simulink library "Library_Drivetrain"  (R2020b)
settings: Solver=VariableStepAuto  StartTime=0.0  StopTime=10.0  RelTol=1e-3
undefined symbols (not defined in the file or in its folder): DrivetrainLeft, DrivetrainRight
libraries: simulink x18, mbd_s32k1xx_ec_toolbox x8
(part 1 of 2)
settings Model: Creator=cbeal  LastModifiedBy=cbeal

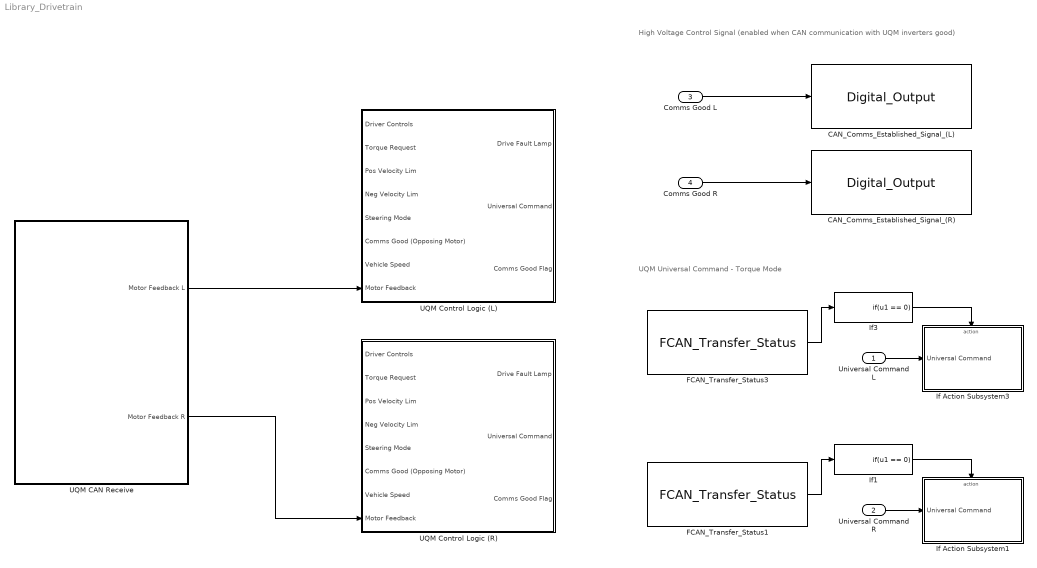
== system Library_Drivetrain ==
  note: UQM Universal Command - Torque Mode
  note: High Voltage Control Signal
      | (enabled when CAN communication with UQM inverters good)
  Universal Command L : Inport
  Universal Command R : Inport  Port=2
  Comms Good L : Inport  Port=3
  Comms Good R : Inport  Port=4
  CAN_Comms_Established_Signal_(L) : mbd_s32k1xx_ec_toolbox/GPIO Blocks/Digital_Output  gpio_pin=PTD8: [PTD8 | Port D I/O]  init_val=Low  drive_strength=Low
  CAN_Comms_Established_Signal_(R) : mbd_s32k1xx_ec_toolbox/GPIO Blocks/Digital_Output  gpio_pin=PTE15: [PTE15 | Port E I/O]  init_val=Low  drive_strength=Low
  FCAN_Transfer_Status1 : mbd_s32k1xx_ec_toolbox/Communication Blocks/CAN Blocks/FCAN_Transfer_Status  can_instance=1  can_mb_idx=4
  FCAN_Transfer_Status3 : mbd_s32k1xx_ec_toolbox/Communication Blocks/CAN Blocks/FCAN_Transfer_Status  can_instance=1  can_mb_idx=3
  If Action Subsystem1 : Subsystem  TreatAsAtomicUnit=on
  If Action Subsystem3 : Subsystem  TreatAsAtomicUnit=on
  If1 : If  IfExpression=u1 == 0  ShowElse=off
  If3 : If  IfExpression=u1 == 0  ShowElse=off
  UQM CAN Receive : Subsystem
  UQM Control Logic (L) : Subsystem  TreatAsAtomicUnit=on
      settings: RTWSystemCode=Inline
  UQM Control Logic (R) : Subsystem  TreatAsAtomicUnit=on
      settings: RTWSystemCode=Inline
  wires:
  UQM CAN Receive/1(Motor Feedback L) -> UQM Control Logic (L)/8(Motor Feedback)
  UQM CAN Receive/2(Motor Feedback R) -> UQM Control Logic (R)/8(Motor Feedback)
  Universal Command L/1 -> If Action Subsystem3/1(Universal Command)
  Universal Command R/1 -> If Action Subsystem1/1(Universal Command)
  If1/1 -> If Action Subsystem1/Action
  If3/1 -> If Action Subsystem3/Action
  FCAN_Transfer_Status3/1 -> If3/1
  FCAN_Transfer_Status1/1 -> If1/1
  Comms Good R/1 -> CAN_Comms_Established_Signal_(R)/1
  Comms Good L/1 -> CAN_Comms_Established_Signal_(L)/1

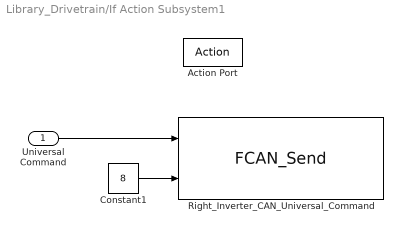
== system Library_Drivetrain/If Action Subsystem1 ==
  Universal Command : Inport
  Action Port : ActionPort  ActionPortLabel=if(u1 == 0)
  Constant1 : Constant  Value=8  OutDataTypeStr=Inherit: Inherit via back propagation
  Right_Inverter_CAN_Universal_Command : mbd_s32k1xx_ec_toolbox/Communication Blocks/CAN Blocks/FCAN_Send  can_instance=1  can_mode=Non-blocking  can_timeout_ms=0  can_mb_idx=4  can_extended_id=off  can_is_remote=off  can_id=F5  show_adv_opts=off  can_fd_enable=off  can_enable_brs=off  can_fd_padding=0
  wires:
  Constant1/1 -> Right_Inverter_CAN_Universal_Command/2
  Universal Command/1 -> Right_Inverter_CAN_Universal_Command/1

== system Library_Drivetrain/If Action Subsystem3 ==
  Universal Command : Inport
  Action Port : ActionPort  ActionPortLabel=if(u1 == 0)
  Constant1 : Constant  Value=8  OutDataTypeStr=Inherit: Inherit via back propagation
  Left_Inverter_CAN_Universal_Command : mbd_s32k1xx_ec_toolbox/Communication Blocks/CAN Blocks/FCAN_Send  can_instance=1  can_mode=Non-blocking  can_timeout_ms=0  can_mb_idx=3  can_extended_id=off  can_is_remote=off  can_id=85  show_adv_opts=off  can_fd_enable=off  can_enable_brs=off  can_fd_padding=0
  wires:
  Universal Command/1 -> Left_Inverter_CAN_Universal_Command/1
  Constant1/1 -> Left_Inverter_CAN_Universal_Command/2

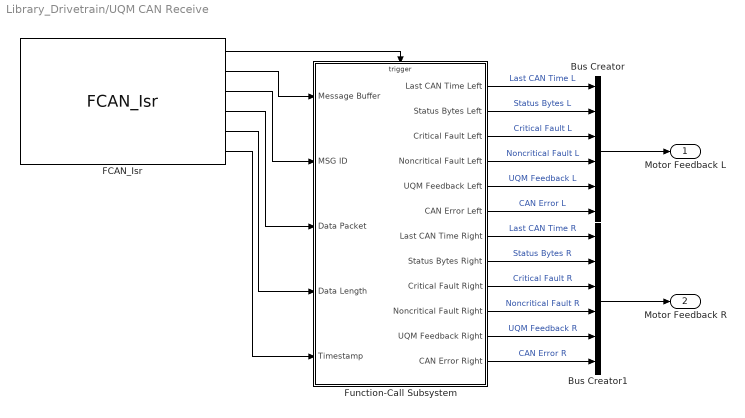
== system Library_Drivetrain/UQM CAN Receive ==
  Bus Creator : BusCreator  Inputs=6
  Bus Creator1 : BusCreator  Inputs=6
  FCAN_Isr : mbd_s32k1xx_ec_toolbox/Communication Blocks/CAN Blocks/FCAN_Isr  can_instance=1  can_event=Rx Complete
  Function-Call Subsystem : Subsystem  TreatAsAtomicUnit=on
  Motor Feedback L : Outport
  Motor Feedback R : Outport  Port=2
  wires:
  FCAN_Isr/2 -> Function-Call Subsystem/1(Message Buffer)
  FCAN_Isr/5 -> Function-Call Subsystem/4(Data Length)
  FCAN_Isr/4 -> Function-Call Subsystem/3(Data Packet)
  FCAN_Isr/3 -> Function-Call Subsystem/2(MSG ID)
  FCAN_Isr/1 -> Function-Call Subsystem/Trigger
  FCAN_Isr/6 -> Function-Call Subsystem/5(Timestamp)
  Function-Call Subsystem/1(Last CAN Time Left) -> Bus Creator/1  "Last CAN Time L"
  Function-Call Subsystem/2(Status Bytes Left) -> Bus Creator/2  "Status Bytes L"
  Function-Call Subsystem/3(Critical Fault Left) -> Bus Creator/3  "Critical Fault L"
  Function-Call Subsystem/4(Noncritical Fault Left) -> Bus Creator/4  "Noncritical Fault L"
  Function-Call Subsystem/5(UQM Feedback Left) -> Bus Creator/5  "UQM Feedback L"
  Function-Call Subsystem/6(CAN Error Left) -> Bus Creator/6  "CAN Error L"
  Bus Creator/1 -> Motor Feedback L/1
  Function-Call Subsystem/7(Last CAN Time Right) -> Bus Creator1/1  "Last CAN Time R"
  Function-Call Subsystem/8(Status Bytes Right) -> Bus Creator1/2  "Status Bytes R"
  Function-Call Subsystem/9(Critical Fault Right) -> Bus Creator1/3  "Critical Fault R"
  Function-Call Subsystem/10(Noncritical Fault Right) -> Bus Creator1/4  "Noncritical Fault R"
  Function-Call Subsystem/11(UQM Feedback Right) -> Bus Creator1/5  "UQM Feedback R"
  Function-Call Subsystem/12(CAN Error Right) -> Bus Creator1/6  "CAN Error R"
  Bus Creator1/1 -> Motor Feedback R/1

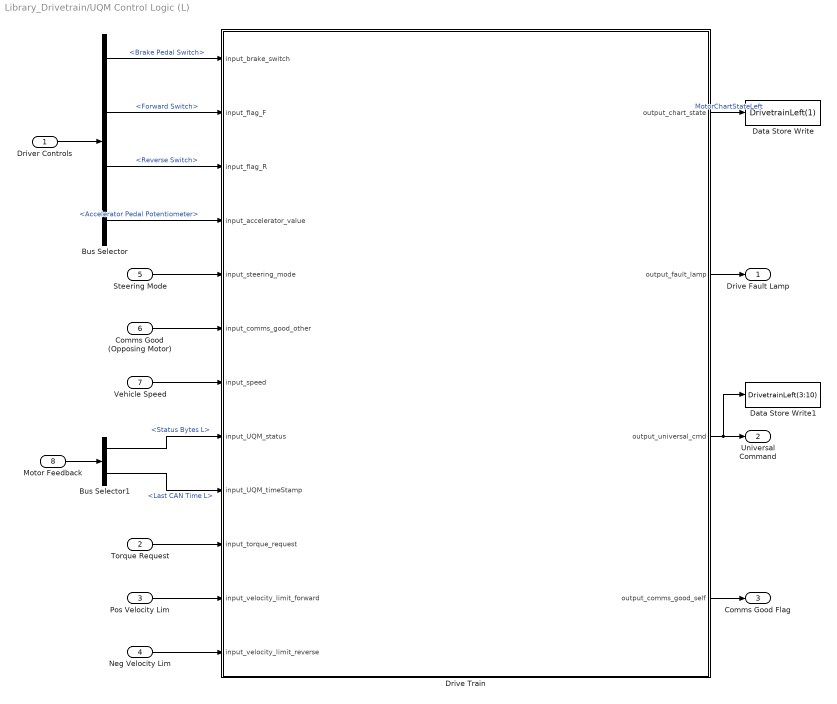
== system Library_Drivetrain/UQM Control Logic (L) ==
  Driver Controls : Inport
  Torque Request : Inport  Port=2
  Pos Velocity Lim : Inport  Port=3
  Neg Velocity Lim : Inport  Port=4
  Steering Mode : Inport  Port=5
  Comms Good (Opposing Motor) : Inport  Port=6
  Vehicle Speed : Inport  Port=7
  Motor Feedback : Inport  Port=8
  Bus Selector : BusSelector  OutputSignals=Brake Pedal Switch,Forward Switch,Reverse Switch,Accelerator Pedal Potentiometer
  Bus Selector1 : BusSelector  OutputSignals=Status Bytes L,Last CAN Time L
  Data Store Write : DataStoreWrite  DataStoreName=DrivetrainLeft  DataStoreElements=DrivetrainLeft(1)
  Data Store Write1 : DataStoreWrite  DataStoreName=DrivetrainLeft  DataStoreElements=DrivetrainLeft(3:10)
  Drive Train : Stateflow chart  TreatAsAtomicUnit=on
      settings: RTWSystemCode=Inline  PortSchema="{\"entries\":[{\"content\":{\"sides\":[{\"content\":{\"connectorIds\":[\"In1\",\"In6\",\"In7\",\"In5\",\"In3\",\"In2\",\"In4\",\"In8\",\"In9\",\"In10\",\"In11\",\"In12\"]},\"type\":\"ConnectorPlacement.EquallySpacedRectSide\",\"uuid\":\"177131f9-522e-4b0e-bcb9-1c7f9e428ff0\"},{\"content\":{\"connectorIds\":[\"Out1\",\"Out2\",\"Out3\",\"Out4\"],\"side\":\"RIGHT\"},\"type\":\"ConnectorPlacement.EquallySpacedRectSide\",\"uuid\":\"9c682759-a653-4ffd-ae7a-9eeda4cc7cea\"},{\"content\":{\"connectorIds\":[],\"side\":\"TOP\"},\"type\":\"ConnectorPlacement.EquallySpacedRectSide\",\"uuid\":\"64c937ee-85b6-4d66-9bbf-f706f379c6d1\"},{\"content\":{\"connectorIds\":[],\"side\":\"HIDDEN\"},\"type\":\"ConnectorPlacement.EquallySpacedRectSide\",\"uuid\":\"ab261037-f33d-4213-8477-31b1a1e7b9c4\"}]},\"type\":\"ConnectorPlacement.EquallySpacedConnector\",\"uuid\":\"dccf0cbc-1b8f-4706-82c8-4b900e553059\"}],\"packageUris\":[\"http://schema.mathworks.com/mf0/Connector/R2020b\"],\"version\":\"1.0\"}"
  Drive Fault Lamp : Outport
  Universal Command : Outport  Port=2
  Comms Good Flag : Outport  Port=3
  wires:
  Drive Train/1(output_chart_state) -> Data Store Write/1  "MotorChartStateLeft"
  Drive Train/3(output_universal_cmd) -> Data Store Write1/1, Universal Command/1
  Drive Train/4(output_comms_good_self) -> Comms Good Flag/1
  Drive Train/2(output_fault_lamp) -> Drive Fault Lamp/1
  Driver Controls/1 -> Bus Selector/1
  Bus Selector/2 -> Drive Train/6(input_flag_F)  "<Forward Switch>"
  Bus Selector/3 -> Drive Train/7(input_flag_R)  "<Reverse Switch>"
  Bus Selector/1 -> Drive Train/1(input_brake_switch)  "<Brake Pedal Switch>"
  Bus Selector/4 -> Drive Train/5(input_accelerator_value)  "<Accelerator Pedal Potentiometer>"
  Torque Request/1 -> Drive Train/10(input_torque_request)
  Pos Velocity Lim/1 -> Drive Train/11(input_velocity_limit_forward)
  Neg Velocity Lim/1 -> Drive Train/12(input_velocity_limit_reverse)
  Steering Mode/1 -> Drive Train/3(input_steering_mode)
  Comms Good (Opposing Motor)/1 -> Drive Train/2(input_comms_good_other)
  Vehicle Speed/1 -> Drive Train/4(input_speed)
  Bus Selector1/2 -> Drive Train/9(input_UQM_timeStamp)  "<Last CAN Time L>"
  Bus Selector1/1 -> Drive Train/8(input_UQM_status)  "<Status Bytes L>"
  Motor Feedback/1 -> Bus Selector1/1

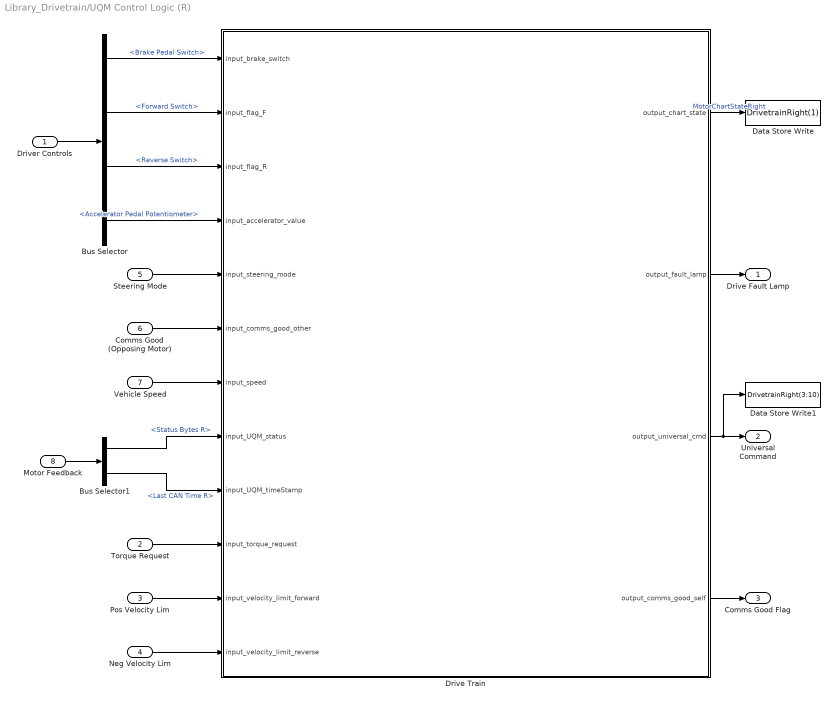
== system Library_Drivetrain/UQM Control Logic (R) ==
  Driver Controls : Inport
  Torque Request : Inport  Port=2
  Pos Velocity Lim : Inport  Port=3
  Neg Velocity Lim : Inport  Port=4
  Steering Mode : Inport  Port=5
  Comms Good (Opposing Motor) : Inport  Port=6
  Vehicle Speed : Inport  Port=7
  Motor Feedback : Inport  Port=8
  Bus Selector : BusSelector  OutputSignals=Brake Pedal Switch,Forward Switch,Reverse Switch,Accelerator Pedal Potentiometer
  Bus Selector1 : BusSelector  OutputSignals=Status Bytes R,Last CAN Time R
  Data Store Write : DataStoreWrite  DataStoreName=DrivetrainRight  DataStoreElements=DrivetrainRight(1)
  Data Store Write1 : DataStoreWrite  DataStoreName=DrivetrainRight  DataStoreElements=DrivetrainRight(3:10)
  Drive Train : Stateflow chart  TreatAsAtomicUnit=on
      settings: RTWSystemCode=Inline  PortSchema="{\"entries\":[{\"content\":{\"sides\":[{\"content\":{\"connectorIds\":[\"In1\",\"In6\",\"In7\",\"In5\",\"In3\",\"In2\",\"In4\",\"In8\",\"In9\",\"In10\",\"In11\",\"In12\"]},\"type\":\"ConnectorPlacement.EquallySpacedRectSide\",\"uuid\":\"177131f9-522e-4b0e-bcb9-1c7f9e428ff0\"},{\"content\":{\"connectorIds\":[\"Out1\",\"Out2\",\"Out3\",\"Out4\"],\"side\":\"RIGHT\"},\"type\":\"ConnectorPlacement.EquallySpacedRectSide\",\"uuid\":\"9c682759-a653-4ffd-ae7a-9eeda4cc7cea\"},{\"content\":{\"connectorIds\":[],\"side\":\"TOP\"},\"type\":\"ConnectorPlacement.EquallySpacedRectSide\",\"uuid\":\"64c937ee-85b6-4d66-9bbf-f706f379c6d1\"},{\"content\":{\"connectorIds\":[],\"side\":\"HIDDEN\"},\"type\":\"ConnectorPlacement.EquallySpacedRectSide\",\"uuid\":\"ab261037-f33d-4213-8477-31b1a1e7b9c4\"}]},\"type\":\"ConnectorPlacement.EquallySpacedConnector\",\"uuid\":\"dccf0cbc-1b8f-4706-82c8-4b900e553059\"}],\"packageUris\":[\"http://schema.mathworks.com/mf0/Connector/R2020b\"],\"version\":\"1.0\"}"
  Drive Fault Lamp : Outport
  Universal Command : Outport  Port=2
  Comms Good Flag : Outport  Port=3
  wires:
  Motor Feedback/1 -> Bus Selector1/1
  Bus Selector1/1 -> Drive Train/8(input_UQM_status)  "<Status Bytes R>"
  Bus Selector1/2 -> Drive Train/9(input_UQM_timeStamp)  "<Last CAN Time R>"
  Vehicle Speed/1 -> Drive Train/4(input_speed)
  Comms Good (Opposing Motor)/1 -> Drive Train/2(input_comms_good_other)
  Steering Mode/1 -> Drive Train/3(input_steering_mode)
  Neg Velocity Lim/1 -> Drive Train/12(input_velocity_limit_reverse)
  Pos Velocity Lim/1 -> Drive Train/11(input_velocity_limit_forward)
  Torque Request/1 -> Drive Train/10(input_torque_request)
  Bus Selector/4 -> Drive Train/5(input_accelerator_value)  "<Accelerator Pedal Potentiometer>"
  Bus Selector/1 -> Drive Train/1(input_brake_switch)  "<Brake Pedal Switch>"
  Bus Selector/3 -> Drive Train/7(input_flag_R)  "<Reverse Switch>"
  Bus Selector/2 -> Drive Train/6(input_flag_F)  "<Forward Switch>"
  Driver Controls/1 -> Bus Selector/1
  Drive Train/2(output_fault_lamp) -> Drive Fault Lamp/1
  Drive Train/4(output_comms_good_self) -> Comms Good Flag/1
  Drive Train/3(output_universal_cmd) -> Universal Command/1, Data Store Write1/1
  Drive Train/1(output_chart_state) -> Data Store Write/1  "MotorChartStateRight"

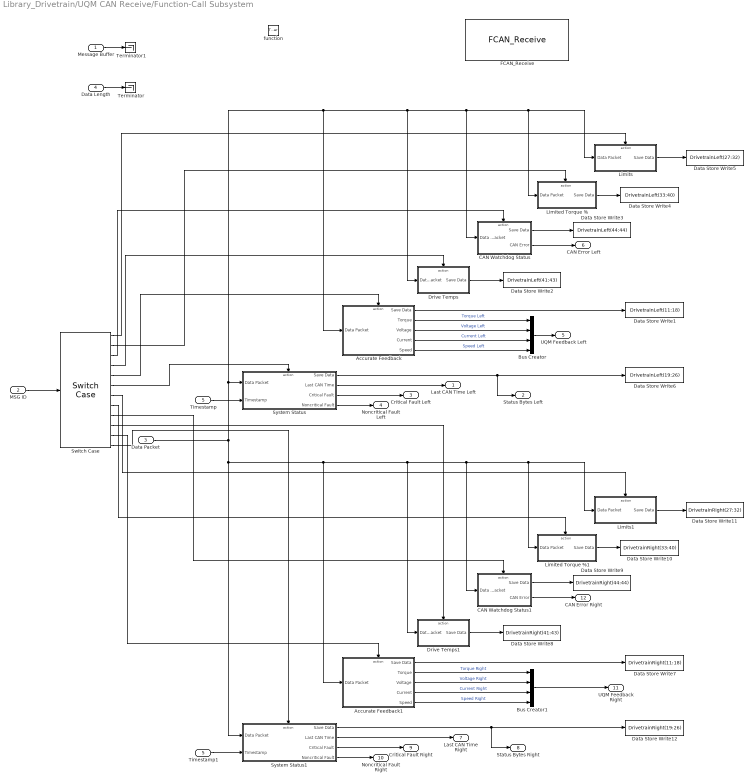
== system Library_Drivetrain/UQM CAN Receive/Function-Call Subsystem ==
  Message Buffer : Inport
  MSG ID : Inport  Port=2
  Data Packet : Inport  Port=3
  Data Length : Inport  Port=4
  Timestamp : Inport  Port=5
  function : TriggerPort  TriggerType=function-call  VariantControl=Variant
  Accurate Feedback : Subsystem  TreatAsAtomicUnit=on
      settings: RTWSystemCode=Inline
  Accurate Feedback1 : Subsystem  TreatAsAtomicUnit=on
      settings: RTWSystemCode=Inline
  Bus Creator : BusCreator  Inputs=4
  Bus Creator1 : BusCreator  Inputs=4
  CAN Watchdog Status : Subsystem  TreatAsAtomicUnit=on
      settings: RTWSystemCode=Inline
  CAN Watchdog Status1 : Subsystem  TreatAsAtomicUnit=on
      settings: RTWSystemCode=Inline
  Data Store Write1 : DataStoreWrite  DataStoreName=DrivetrainLeft  DataStoreElements=DrivetrainLeft(11:18)
  Data Store Write10 : DataStoreWrite  DataStoreName=DrivetrainRight  DataStoreElements=DrivetrainRight(33:40)
  Data Store Write11 : DataStoreWrite  DataStoreName=DrivetrainRight  DataStoreElements=DrivetrainRight(27:32)
  Data Store Write12 : DataStoreWrite  DataStoreName=DrivetrainRight  DataStoreElements=DrivetrainRight(19:26)
  Data Store Write2 : DataStoreWrite  DataStoreName=DrivetrainLeft  DataStoreElements=DrivetrainLeft(41:43)
  Data Store Write3 : DataStoreWrite  DataStoreName=DrivetrainLeft  DataStoreElements=DrivetrainLeft(44:44)
  Data Store Write4 : DataStoreWrite  DataStoreName=DrivetrainLeft  DataStoreElements=DrivetrainLeft(33:40)
  Data Store Write5 : DataStoreWrite  DataStoreName=DrivetrainLeft  DataStoreElements=DrivetrainLeft(27:32)
  Data Store Write6 : DataStoreWrite  DataStoreName=DrivetrainLeft  DataStoreElements=DrivetrainLeft(19:26)
  Data Store Write7 : DataStoreWrite  DataStoreName=DrivetrainRight  DataStoreElements=DrivetrainRight(11:18)
  Data Store Write8 : DataStoreWrite  DataStoreName=DrivetrainRight  DataStoreElements=DrivetrainRight(41:43)
  Data Store Write9 : DataStoreWrite  DataStoreName=DrivetrainRight  DataStoreElements=DrivetrainRight(44:44)
  Drive Temps : Subsystem  TreatAsAtomicUnit=on
      settings: RTWSystemCode=Inline
  Drive Temps1 : Subsystem  TreatAsAtomicUnit=on
      settings: RTWSystemCode=Inline
  FCAN_Receive : mbd_s32k1xx_ec_toolbox/Communication Blocks/CAN Blocks/FCAN_Receive  can_instance=1  can_mode=Non-blocking  can_timeout_ms=0  can_mb_idx=0  can_extended_id=off  can_is_remote=off  can_id=0  can_msg_mask=0  show_adv_opts=off  can_use_rxfifo=off  can_fd_enable=off
  Limited Torque % : Subsystem  TreatAsAtomicUnit=on
      settings: RTWSystemCode=Inline
  Limited Torque %1 : Subsystem  TreatAsAtomicUnit=on
      settings: RTWSystemCode=Inline
  Limits : Subsystem  TreatAsAtomicUnit=on
      settings: RTWSystemCode=Inline
  Limits1 : Subsystem  TreatAsAtomicUnit=on
      settings: RTWSystemCode=Inline
  Switch Case : SwitchCase  CaseConditions={hex2dec('8C'),hex2dec('8D'),hex2dec('8F'),hex2dec('8E'),hex2dec('89'),hex2dec('8A'),hex2dec('FC'),hex2dec('FD'),hex2dec('FF'),hex2dec('FE'),hex2dec('F9'),hex2dec('FA')}  ShowDefaultCase=off
  System Status : Subsystem  TreatAsAtomicUnit=on
      settings: RTWSystemCode=Inline
  System Status1 : Subsystem  TreatAsAtomicUnit=on
      settings: RTWSystemCode=Inline
  Terminator : Terminator
  Terminator1 : Terminator
  Timestamp1 : InportShadow  Port=5
  Last CAN Time Left : Outport
  Status Bytes Left : Outport  Port=2
  Critical Fault Left : Outport  Port=3
  Noncritical Fault Left : Outport  Port=4
  UQM Feedback Left : Outport  Port=5
  CAN Error Left : Outport  Port=6
  Last CAN Time Right : Outport  Port=7
  Status Bytes Right : Outport  Port=8
  Critical Fault Right : Outport  Port=9
  Noncritical Fault Right : Outport  Port=10
  UQM Feedback Right : Outport  Port=11
  CAN Error Right : Outport  Port=12
  wires:
  Drive Temps/1(Save Data) -> Data Store Write2/1
  CAN Watchdog Status/1(Save Data) -> Data Store Write3/1
  System Status/1(Save Data) -> Data Store Write6/1, Status Bytes Left/1
  Switch Case/2 -> Limited Torque %/Action
  Switch Case/4 -> Drive Temps/Action
  Switch Case/3 -> CAN Watchdog Status/Action
  Accurate Feedback/3(Voltage) -> Bus Creator/2  "Voltage Left"
  MSG ID/1 -> Switch Case/1
  Timestamp/1 -> System Status/2(Timestamp)
  System Status/4(Noncritical Fault) -> Noncritical Fault Left/1
  Message Buffer/1 -> Terminator1/1
  System Status/3(Critical Fault) -> Critical Fault Left/1
  CAN Watchdog Status/2(CAN Error) -> CAN Error Left/1
  Switch Case/1 -> Limits/Action
  Bus Creator/1 -> UQM Feedback Left/1
  Data Length/1 -> Terminator/1
  Switch Case/6 -> System Status/Action
  Accurate Feedback/5(Speed) -> Bus Creator/4  "Speed Left"
  Switch Case/5 -> Accurate Feedback/Action
  System Status/2(Last CAN Time) -> Last CAN Time Left/1
  Accurate Feedback/4(Current) -> Bus Creator/3  "Current Left"
  Limits/1(Save Data) -> Data Store Write5/1
  Accurate Feedback/1(Save Data) -> Data Store Write1/1
  Limited Torque %/1(Save Data) -> Data Store Write4/1
  Accurate Feedback/2(Torque) -> Bus Creator/1  "Torque Left"
  Limited Torque %1/1(Save Data) -> Data Store Write10/1
  Accurate Feedback1/2(Torque) -> Bus Creator1/1  "Torque Right"
  Accurate Feedback1/1(Save Data) -> Data Store Write7/1
  Limits1/1(Save Data) -> Data Store Write11/1
  System Status1/2(Last CAN Time) -> Last CAN Time Right/1
  Switch Case/12 -> System Status1/Action
  Switch Case/11 -> Accurate Feedback1/Action
  System Status1/3(Critical Fault) -> Critical Fault Right/1
  Data Packet/1 -> Accurate Feedback1/1(Data Packet), Drive Temps1/1(Data Packet), CAN Watchdog Status1/1(Data Packet), Limited Torque %1/1(Data Packet), Limits1/1(Data Packet), System Status1/1(Data Packet), Accurate Feedback/1(Data Packet), Drive Temps/1(Data Packet), CAN Watchdog Status/1(Data Packet), Limited Torque %/1(Data Packet), Limits/1(Data Packet), System Status/1(Data Packet)
  Bus Creator1/1 -> UQM Feedback Right/1
  Switch Case/10 -> Drive Temps1/Action
  Accurate Feedback1/4(Current) -> Bus Creator1/3  "Current Right"
  Switch Case/9 -> CAN Watchdog Status1/Action
  Accurate Feedback1/5(Speed) -> Bus Creator1/4  "Speed Right"
  Drive Temps1/1(Save Data) -> Data Store Write8/1
  CAN Watchdog Status1/1(Save Data) -> Data Store Write9/1
  System Status1/4(Noncritical Fault) -> Noncritical Fault Right/1
  System Status1/1(Save Data) -> Data Store Write12/1, Status Bytes Right/1
  Switch Case/7 -> Limits1/Action
  Accurate Feedback1/3(Voltage) -> Bus Creator1/2  "Voltage Right"
  Timestamp1/1 -> System Status1/2(Timestamp)
  Switch Case/8 -> Limited Torque %1/Action
  CAN Watchdog Status1/2(CAN Error) -> CAN Error Right/1

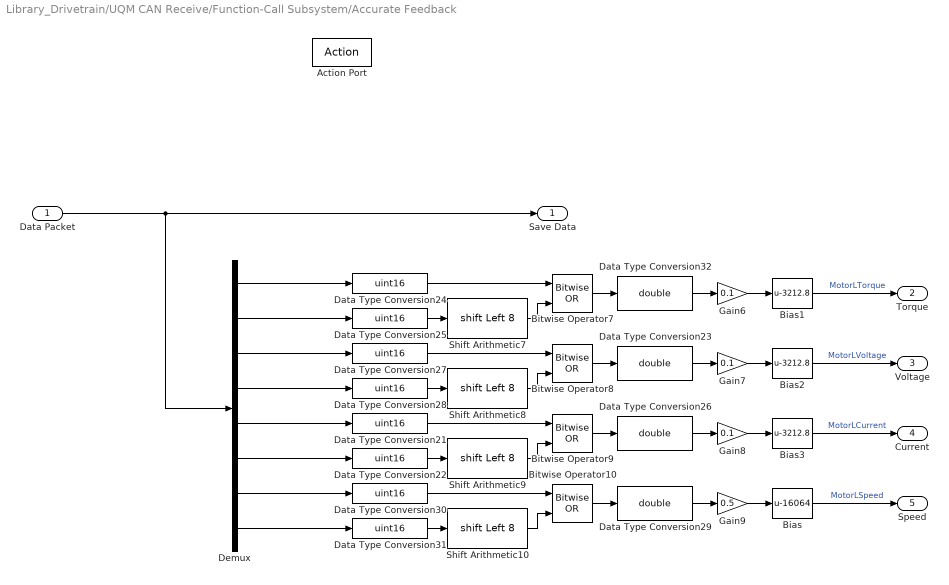
== system Library_Drivetrain/UQM CAN Receive/Function-Call Subsystem/Accurate Feedback ==
  Data Packet : Inport
  Action Port : ActionPort
  Bias : Bias  Bias=-16064
  Bias1 : Bias  Bias=-3212.8
  Bias2 : Bias  Bias=-3212.8
  Bias3 : Bias  Bias=-3212.8
  Bitwise Operator{7..10} (4 alike) : simulink/Logic and Bit Operations/Bitwise Operator  logicop=OR  UseBitMask=off  NumInputPorts=2  BitMask=bin2dec('11011001')  BitMaskRealWorld=Stored Integer
  Data Type Conversion{21..22,24..25,27..28,30..31} (8 alike) : DataTypeConversion  OutDataTypeStr=uint16
  Data Type Conversion{23,26,29,32} (4 alike) : DataTypeConversion  OutDataTypeStr=double
  Demux : Demux  Outputs=8
  Gain6 : Gain  Gain=0.1  OutDataTypeStr=Inherit: Inherit via back propagation
  Gain7 : Gain  Gain=0.1  OutDataTypeStr=Inherit: Inherit via back propagation
  Gain8 : Gain  Gain=0.1  OutDataTypeStr=Inherit: Inherit via back propagation
  Gain9 : Gain  Gain=0.5  OutDataTypeStr=Inherit: Inherit via back propagation
  Shift Arithmetic{7..10} (4 alike) : ArithShift  BitShiftNumber=8  BitShiftDirection=Left
  Save Data : Outport
  Torque : Outport  Port=2
  Voltage : Outport  Port=3
  Current : Outport  Port=4
  Speed : Outport  Port=5
  wires:
  Bias1/1 -> Torque/1  "MotorLTorque"
  Bias2/1 -> Voltage/1  "MotorLVoltage"
  Bias3/1 -> Current/1  "MotorLCurrent"
  Bias/1 -> Speed/1  "MotorLSpeed"
  Data Type Conversion24/1 -> Bitwise Operator7/1
  Gain7/1 -> Bias2/1
  Data Type Conversion30/1 -> Bitwise Operator10/1
  Data Type Conversion22/1 -> Shift Arithmetic9/1
  Data Type Conversion21/1 -> Bitwise Operator9/1
  Bitwise Operator9/1 -> Data Type Conversion26/1
  Gain9/1 -> Bias/1
  Data Type Conversion28/1 -> Shift Arithmetic8/1
  Data Type Conversion32/1 -> Gain6/1
  Shift Arithmetic7/1 -> Bitwise Operator7/2
  Gain8/1 -> Bias3/1
  Data Type Conversion26/1 -> Gain8/1
  Bitwise Operator10/1 -> Data Type Conversion29/1
  Bitwise Operator8/1 -> Data Type Conversion23/1
  Gain6/1 -> Bias1/1
  Shift Arithmetic10/1 -> Bitwise Operator10/2
  Data Type Conversion27/1 -> Bitwise Operator8/1
  Data Type Conversion29/1 -> Gain9/1
  Bitwise Operator7/1 -> Data Type Conversion32/1
  Data Type Conversion31/1 -> Shift Arithmetic10/1
  Data Type Conversion25/1 -> Shift Arithmetic7/1
  Shift Arithmetic8/1 -> Bitwise Operator8/2
  Shift Arithmetic9/1 -> Bitwise Operator9/2
  Data Type Conversion23/1 -> Gain7/1
  Demux/1 -> Data Type Conversion24/1
  Demux/2 -> Data Type Conversion25/1
  Demux/3 -> Data Type Conversion27/1
  Demux/4 -> Data Type Conversion28/1
  Demux/5 -> Data Type Conversion21/1
  Demux/6 -> Data Type Conversion22/1
  Demux/7 -> Data Type Conversion30/1
  Demux/8 -> Data Type Conversion31/1
  Data Packet/1 -> Demux/1, Save Data/1

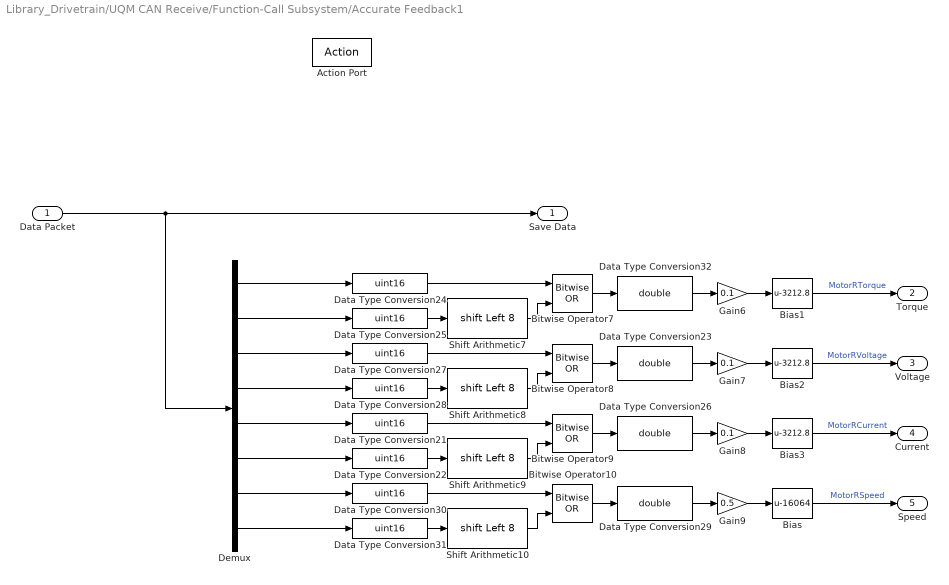
== system Library_Drivetrain/UQM CAN Receive/Function-Call Subsystem/Accurate Feedback1 ==
  Data Packet : Inport
  Action Port : ActionPort
  Bias : Bias  Bias=-16064
  Bias1 : Bias  Bias=-3212.8
  Bias2 : Bias  Bias=-3212.8
  Bias3 : Bias  Bias=-3212.8
  Bitwise Operator{7..10} (4 alike) : simulink/Logic and Bit Operations/Bitwise Operator  logicop=OR  UseBitMask=off  NumInputPorts=2  BitMask=bin2dec('11011001')  BitMaskRealWorld=Stored Integer
  Data Type Conversion{21..22,24..25,27..28,30..31} (8 alike) : DataTypeConversion  OutDataTypeStr=uint16
  Data Type Conversion{23,26,29,32} (4 alike) : DataTypeConversion  OutDataTypeStr=double
  Demux : Demux  Outputs=8
  Gain6 : Gain  Gain=0.1  OutDataTypeStr=Inherit: Inherit via back propagation
  Gain7 : Gain  Gain=0.1  OutDataTypeStr=Inherit: Inherit via back propagation
  Gain8 : Gain  Gain=0.1  OutDataTypeStr=Inherit: Inherit via back propagation
  Gain9 : Gain  Gain=0.5  OutDataTypeStr=Inherit: Inherit via back propagation
  Shift Arithmetic{7..10} (4 alike) : ArithShift  BitShiftNumber=8  BitShiftDirection=Left
  Save Data : Outport
  Torque : Outport  Port=2
  Voltage : Outport  Port=3
  Current : Outport  Port=4
  Speed : Outport  Port=5
  wires:
  Bias1/1 -> Torque/1  "MotorRTorque"
  Bias2/1 -> Voltage/1  "MotorRVoltage"
  Bias3/1 -> Current/1  "MotorRCurrent"
  Bias/1 -> Speed/1  "MotorRSpeed"
  Data Type Conversion24/1 -> Bitwise Operator7/1
  Gain7/1 -> Bias2/1
  Data Type Conversion30/1 -> Bitwise Operator10/1
  Data Type Conversion22/1 -> Shift Arithmetic9/1
  Data Type Conversion21/1 -> Bitwise Operator9/1
  Bitwise Operator9/1 -> Data Type Conversion26/1
  Gain9/1 -> Bias/1
  Data Type Conversion28/1 -> Shift Arithmetic8/1
  Data Type Conversion32/1 -> Gain6/1
  Shift Arithmetic7/1 -> Bitwise Operator7/2
  Gain8/1 -> Bias3/1
  Data Type Conversion26/1 -> Gain8/1
  Bitwise Operator10/1 -> Data Type Conversion29/1
  Bitwise Operator8/1 -> Data Type Conversion23/1
  Gain6/1 -> Bias1/1
  Shift Arithmetic10/1 -> Bitwise Operator10/2
  Data Type Conversion27/1 -> Bitwise Operator8/1
  Data Type Conversion29/1 -> Gain9/1
  Bitwise Operator7/1 -> Data Type Conversion32/1
  Data Type Conversion31/1 -> Shift Arithmetic10/1
  Data Type Conversion25/1 -> Shift Arithmetic7/1
  Shift Arithmetic8/1 -> Bitwise Operator8/2
  Shift Arithmetic9/1 -> Bitwise Operator9/2
  Data Type Conversion23/1 -> Gain7/1
  Demux/1 -> Data Type Conversion24/1
  Demux/2 -> Data Type Conversion25/1
  Demux/3 -> Data Type Conversion27/1
  Demux/4 -> Data Type Conversion28/1
  Demux/5 -> Data Type Conversion21/1
  Demux/6 -> Data Type Conversion22/1
  Demux/7 -> Data Type Conversion30/1
  Demux/8 -> Data Type Conversion31/1
  Data Packet/1 -> Demux/1, Save Data/1

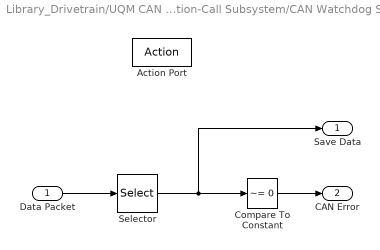
== system Library_Drivetrain/UQM CAN Receive/Function-Call Subsystem/CAN Watchdog Status ==
  Data Packet : Inport
  Action Port : ActionPort
  Compare To Constant : simulink/Logic and Bit Operations/Compare To Constant  relop=~=  const=0  OutDataTypeStr=boolean
  Selector : Selector  InputPortWidth=8  IndexOptions=Index vector (dialog)  Indices=[8]  OutputSizes=1
  Save Data : Outport
  CAN Error : Outport  Port=2
  wires:
  Data Packet/1 -> Selector/1
  Selector/1 -> Save Data/1, Compare To Constant/1
  Compare To Constant/1 -> CAN Error/1

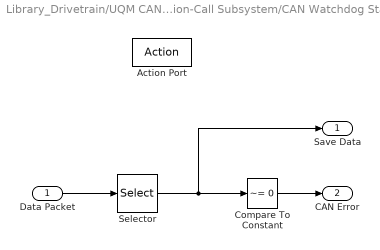
== system Library_Drivetrain/UQM CAN Receive/Function-Call Subsystem/CAN Watchdog Status1 ==
  Data Packet : Inport
  Action Port : ActionPort
  Compare To Constant : simulink/Logic and Bit Operations/Compare To Constant  relop=~=  const=0  OutDataTypeStr=boolean
  Selector : Selector  InputPortWidth=8  IndexOptions=Index vector (dialog)  Indices=[8]  OutputSizes=1
  Save Data : Outport
  CAN Error : Outport  Port=2
  wires:
  Data Packet/1 -> Selector/1
  Selector/1 -> Save Data/1, Compare To Constant/1
  Compare To Constant/1 -> CAN Error/1

== system Library_Drivetrain/UQM CAN Receive/Function-Call Subsystem/Drive Temps ==
  Data Packet : Inport
  Action Port : ActionPort
  Selector : Selector  InputPortWidth=8  IndexOptions=Index vector (dialog)  Indices=[2:4]  OutputSizes=1
  Save Data : Outport
  wires:
  Data Packet/1 -> Selector/1
  Selector/1 -> Save Data/1

== system Library_Drivetrain/UQM CAN Receive/Function-Call Subsystem/Drive Temps1 ==
  Data Packet : Inport
  Action Port : ActionPort
  Selector : Selector  InputPortWidth=8  IndexOptions=Index vector (dialog)  Indices=[2:4]  OutputSizes=1
  Save Data : Outport
  wires:
  Data Packet/1 -> Selector/1
  Selector/1 -> Save Data/1

== system Library_Drivetrain/UQM CAN Receive/Function-Call Subsystem/Limited Torque % ==
  Data Packet : Inport
  Action Port : ActionPort
  Save Data : Outport
  wires:
  Data Packet/1 -> Save Data/1

== system Library_Drivetrain/UQM CAN Receive/Function-Call Subsystem/Limited Torque %1 ==
  Data Packet : Inport
  Action Port : ActionPort
  Save Data : Outport
  wires:
  Data Packet/1 -> Save Data/1

== system Library_Drivetrain/UQM CAN Receive/Function-Call Subsystem/Limits ==
  Data Packet : Inport
  Action Port : ActionPort
  Selector : Selector  InputPortWidth=8  IndexOptions=Index vector (dialog)  Indices=[3:8]  OutputSizes=1
  Save Data : Outport
  wires:
  Data Packet/1 -> Selector/1
  Selector/1 -> Save Data/1

== system Library_Drivetrain/UQM CAN Receive/Function-Call Subsystem/Limits1 ==
  Data Packet : Inport
  Action Port : ActionPort
  Selector : Selector  InputPortWidth=8  IndexOptions=Index vector (dialog)  Indices=[3:8]  OutputSizes=1
  Save Data : Outport
  wires:
  Data Packet/1 -> Selector/1
  Selector/1 -> Save Data/1

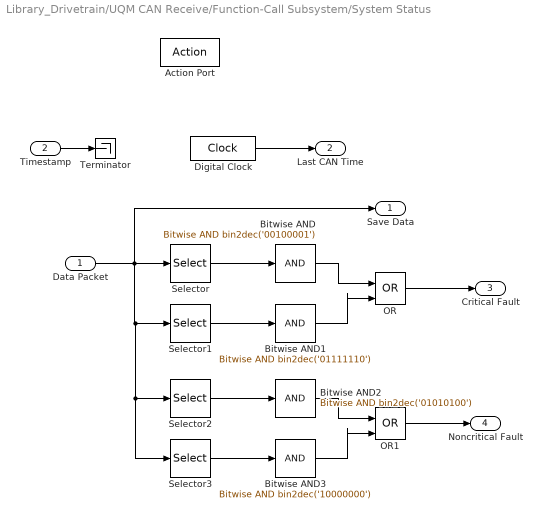
== system Library_Drivetrain/UQM CAN Receive/Function-Call Subsystem/System Status ==
  Data Packet : Inport
  Timestamp : Inport  Port=2
  Action Port : ActionPort
  Bitwise AND : simulink/Logic and Bit Operations/Bitwise Operator  logicop=AND  UseBitMask=on  BitMask=bin2dec('00100001')  BitMaskRealWorld=Stored Integer
  Bitwise AND1 : simulink/Logic and Bit Operations/Bitwise Operator  logicop=AND  UseBitMask=on  BitMask=bin2dec('01111110')  BitMaskRealWorld=Stored Integer
  Bitwise AND2 : simulink/Logic and Bit Operations/Bitwise Operator  logicop=AND  UseBitMask=on  BitMask=bin2dec('01010100')  BitMaskRealWorld=Stored Integer
  Bitwise AND3 : simulink/Logic and Bit Operations/Bitwise Operator  logicop=AND  UseBitMask=on  BitMask=bin2dec('10000000')  BitMaskRealWorld=Stored Integer
  Digital Clock : DigitalClock  SampleTime=-1
  OR : Logic  Operator=OR  IconShape=distinctive  AllPortsSameDT=off  OutDataTypeStr=boolean
  OR1 : Logic  Operator=OR  IconShape=distinctive  AllPortsSameDT=off  OutDataTypeStr=boolean
  Selector : Selector  InputPortWidth=8  IndexOptions=Index vector (dialog)  Indices=7  OutputSizes=1
  Selector1 : Selector  InputPortWidth=8  IndexOptions=Index vector (dialog)  Indices=8  OutputSizes=1
  Selector2 : Selector  InputPortWidth=8  IndexOptions=Index vector (dialog)  Indices=7  OutputSizes=1
  Selector3 : Selector  InputPortWidth=8  IndexOptions=Index vector (dialog)  Indices=8  OutputSizes=1
  Terminator : Terminator
  Save Data : Outport
  Last CAN Time : Outport  Port=2
  Critical Fault : Outport  Port=3
  Noncritical Fault : Outport  Port=4
  wires:
  Data Packet/1 -> Save Data/1, Selector3/1, Selector2/1, Selector1/1, Selector/1
  Selector/1 -> Bitwise AND/1
  Bitwise AND/1 -> OR/1
  OR/1 -> Critical Fault/1
  Selector1/1 -> Bitwise AND1/1
  Bitwise AND1/1 -> OR/2
  Bitwise AND3/1 -> OR1/2
  Selector3/1 -> Bitwise AND3/1
  Bitwise AND2/1 -> OR1/1
  Selector2/1 -> Bitwise AND2/1
  OR1/1 -> Noncritical Fault/1
  Digital Clock/1 -> Last CAN Time/1
  Timestamp/1 -> Terminator/1

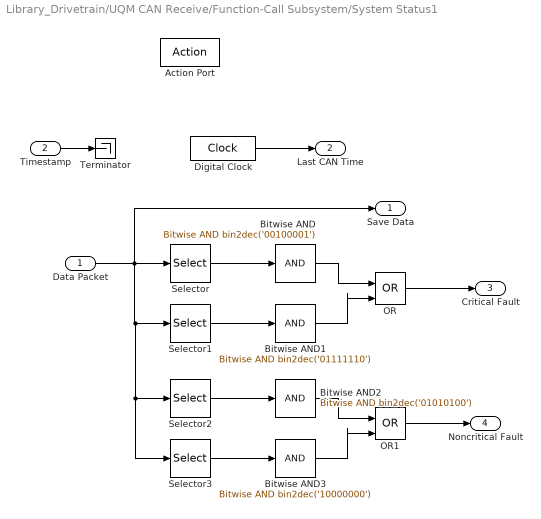
== system Library_Drivetrain/UQM CAN Receive/Function-Call Subsystem/System Status1 ==
  Data Packet : Inport
  Timestamp : Inport  Port=2
  Action Port : ActionPort
  Bitwise AND : simulink/Logic and Bit Operations/Bitwise Operator  logicop=AND  UseBitMask=on  BitMask=bin2dec('00100001')  BitMaskRealWorld=Stored Integer
  Bitwise AND1 : simulink/Logic and Bit Operations/Bitwise Operator  logicop=AND  UseBitMask=on  BitMask=bin2dec('01111110')  BitMaskRealWorld=Stored Integer
  Bitwise AND2 : simulink/Logic and Bit Operations/Bitwise Operator  logicop=AND  UseBitMask=on  BitMask=bin2dec('01010100')  BitMaskRealWorld=Stored Integer
  Bitwise AND3 : simulink/Logic and Bit Operations/Bitwise Operator  logicop=AND  UseBitMask=on  BitMask=bin2dec('10000000')  BitMaskRealWorld=Stored Integer
  Digital Clock : DigitalClock  SampleTime=-1
  OR : Logic  Operator=OR  IconShape=distinctive  AllPortsSameDT=off  OutDataTypeStr=boolean
  OR1 : Logic  Operator=OR  IconShape=distinctive  AllPortsSameDT=off  OutDataTypeStr=boolean
  Selector : Selector  InputPortWidth=8  IndexOptions=Index vector (dialog)  Indices=7  OutputSizes=1
  Selector1 : Selector  InputPortWidth=8  IndexOptions=Index vector (dialog)  Indices=8  OutputSizes=1
  Selector2 : Selector  InputPortWidth=8  IndexOptions=Index vector (dialog)  Indices=7  OutputSizes=1
  Selector3 : Selector  InputPortWidth=8  IndexOptions=Index vector (dialog)  Indices=8  OutputSizes=1
  Terminator : Terminator
  Save Data : Outport
  Last CAN Time : Outport  Port=2
  Critical Fault : Outport  Port=3
  Noncritical Fault : Outport  Port=4
  wires:
  Data Packet/1 -> Save Data/1, Selector3/1, Selector2/1, Selector1/1, Selector/1
  Selector/1 -> Bitwise AND/1
  Bitwise AND/1 -> OR/1
  OR/1 -> Critical Fault/1
  Selector1/1 -> Bitwise AND1/1
  Bitwise AND1/1 -> OR/2
  Bitwise AND3/1 -> OR1/2
  Selector3/1 -> Bitwise AND3/1
  Bitwise AND2/1 -> OR1/1
  Selector2/1 -> Bitwise AND2/1
  OR1/1 -> Noncritical Fault/1
  Digital Clock/1 -> Last CAN Time/1
  Timestamp/1 -> Terminator/1

== stateflow chart Library_Drivetrain/UQM Control Logic (L)/Drive Train ==
  state Drive_Mode [parallel]
    entry:
    universal_cmd_cnt = 0;
    during:
    universal_cmd_cnt = mod(universal_cmd_cnt,16);
    settings: executionOrder=5
    state Normal
      entry:
      output_chart_state = 3;
      during:
      % setting bits 0-3 to torque mode and bits 4-7 to the counter value
      output_universal_cmd(1) = bitor(uint8(1),bitshift(universal_cmd_cnt,4));
      output_universal_cmd(2) = bitor(bitshift(uint8(1),4),bitshift(uint8(input_flag_F),3));
      output_universal_cmd(3:4) = convert_val_to_UQM_CAN_bytes(input_torque_request,-350,350,0.1,3212.8);
      output_universal_cmd(5:6) = convert_val_to_UQM_CAN_bytes(input_velocity_limit_forward,0,5400,0.5,16064);
      output_universal_cmd(7:8) = convert_val_to_UQM_CAN_bytes(input_velocity_limit_reverse,-900,0,0.5,16064);
    state LimitedTorque_LimpHome
      entry:
      output_chart_state = 2;
      % limit what goes out on universal command, override them
      during:
      % setting bits 0-3 to torque mode and bits 4-7 to the counter value
      output_universal_cmd(1) = bitor(uint8(1),bitshift(universal_cmd_cnt,4));
      output_universal_cmd(2) = bitor(bitshift(uint8(1),4),bitshift(uint8(input_flag_F),3));
      output_universal_cmd(3:4) = convert_val_to_UQM_CAN_bytes(input_torque_request,-100,100,0.1,3212.8);
      output_universal_cmd(5:6) = convert_val_to_UQM_CAN_bytes(input_velocity_limit_forward,0,900,0.5,16064);
      output_universal_cmd(7:8) = convert_val_to_UQM_CAN_bytes(input_velocity_limit_reverse,-900,0,0.5,16064);
    state ZeroTorque_Startup
      entry:
      output_chart_state = 1;
      % sending universal command msg (torque/speed limits)
      % completely override for command w zero torque
      during:
      % setting universal command to coast
      output_universal_cmd = uint8([0; 8; hex2dec('80'); hex2dec('7D'); ...
      hex2dec('80'); hex2dec('7D'); hex2dec('80'); hex2dec('7D')]);
      % setting bits 0-3 to torque mode and bits 4-7 to the counter value
      output_universal_cmd(1) = bitor(uint8(1),bitshift(universal_cmd_cnt,4));
    state Shutdown
      entry:
      output_chart_state = 0;
      during:
      % setting universal command to coast
      output_universal_cmd = uint8([0; 8; hex2dec('80'); hex2dec('7D'); ...
      hex2dec('80'); hex2dec('7D'); hex2dec('80'); hex2dec('7D')]);
      % setting bits 0-3 to torque mode and bits 4-7 to the counter value
      output_universal_cmd(1) = bitor(uint8(1),bitshift(universal_cmd_cnt,4));
    Normal -> Shutdown [order 3] : CAN_WD_Timeout
    ZeroTorque_Startup -> Normal [order 3] : [1==input_brake_switch && ...
        | (xor(input_flag_F, input_flag_R)) && ...
        | 1==output_comms_good_self && ...
        | 1==input_comms_good_other && ...
        | 3==input_steering_mode && ...
        | FNR_velocity_match_flag==1 && ...
        | (input_torque_request>-25 && input_torque_request<5)]
        | % negative side might need to be bigger
    Normal -> Shutdown [order 1] : inputs_outside_range
    Normal -> ZeroTorque_Startup [order 4] : [FNR_velocity_match_flag==0]
    Normal -> ZeroTorque_Startup [order 5] : [input_steering_mode==0 || ...
        | input_steering_mode==1]
    Normal -> ZeroTorque_Startup [order 2] : [input_flag_F==0 && ...
        | input_flag_R==0]
    Normal -> LimitedTorque_LimpHome [order 6] : [2==input_steering_mode]
    LimitedTorque_LimpHome -> Normal [order 4] : [1==output_comms_good_self && ...
        | 1==input_comms_good_other && ...
        | 3==input_steering_mode && ...
        | FNR_velocity_match_flag==1 && ...
        | (input_torque_request>-100 && input_torque_request<100)]
        | % negative side might need to be bigger
    LimitedTorque_LimpHome -> Shutdown [order 3] : CAN_WD_Timeout
    LimitedTorque_LimpHome -> Shutdown [order 1] : inputs_outside_range
    LimitedTorque_LimpHome -> ZeroTorque_Startup [order 2] : [(input_flag_F==0 && ...
        | input_flag_R==0) || ...
        | 1==input_steering_mode || ...
        | 0==input_steering_mode]
    ZeroTorque_Startup -> LimitedTorque_LimpHome [order 1] : [1==input_brake_switch && ...
        | (xor(input_flag_F, input_flag_R)) && ...
        | ( ((0==output_comms_good_self && 1==input_comms_good_other) || (1==output_comms_good_self && 0==input_comms_good_other)) || ...
        | (1==output_comms_good_self && 1==input_comms_good_other && 2==input_steering_mode && FNR_velocity_match_flag==1) ) && ...
        | (input_torque_request>-25 && input_torque_request<5)]
        | % negative side might need to be bigger
    (default) -> ZeroTorque_Startup
    ZeroTorque_Startup -> Shutdown [order 4] : CAN_WD_Timeout
    ZeroTorque_Startup -> Shutdown [order 2] : inputs_outside_range
  state Fault_Lamp_Control [parallel]
    settings: executionOrder=6
    state Steady_OFF
      during:
      output_fault_lamp = 0;
    state Blink_OFF
      during:
      output_fault_lamp = 0;
    state Blink_ON
      during:
      output_fault_lamp = 1;
    state Steady_ON
      during:
      output_fault_lamp = 1;
    Steady_OFF -> Fault_Lamp_Control : [output_chart_state ~= 3]
    (junction 373) -> Steady_OFF [order 2] : [output_chart_state == 3]
    Blink_ON -> Steady_OFF [order 1] : [output_chart_state == 3]
    Blink_OFF -> Steady_OFF [order 1] : [output_chart_state == 3]
    Blink_OFF -> Blink_ON [order 3] : [elapsed > double(output_chart_state)*0.2]
    (default) -> (junction 373)
    (junction 373) -> Blink_ON [order 3]
    (junction 373) -> Steady_ON [order 1] : [output_chart_state == 0]
    Blink_ON -> Blink_OFF [order 3] : [elapsed > double(output_chart_state)*0.2]
    Blink_ON -> Steady_ON [order 2] : [output_chart_state == 0]
    Blink_OFF -> Steady_ON [order 2] : [output_chart_state == 0]
    Steady_ON -> Fault_Lamp_Control : [output_chart_state ~= 0]
  state CAN_Watchdog [parallel]
    entry:
    lastUQMWatchDogTime = 0;
    output_comms_good_self = false;
    settings: executionOrder=1
    state CAN_Good
    state CAN_Lost
      entry:
      output_comms_good_self=false;
    (default) -> CAN_Good
    CAN_Good -> CAN_Watchdog [order 2] : [input_UQM_timeStamp ~= lastUQMWatchDogTime]...
        | {lastUQMWatchDogTime = input_UQM_timeStamp; output_comms_good_self=true}
    CAN_Good -> CAN_Lost [order 1] : [elapsed > 1.2 && lastUQMWatchDogTime ~= 0] {send(CAN_WD_Timeout, Drive_Mode)}
  state Input_check [parallel]
    during:
    settings: executionOrder=4
    state Input_check_if_statement
      (default) -> (junction 279)
      (junction 279) -> (junction 280) [order 1] : [input_velocity_limit_forward>5400 || ...
          | input_velocity_limit_forward<0]
      (junction 279) -> (junction 266) [order 2]
      (junction 280) -> (junction 281)
      (junction 266) -> (junction 269) [order 1] : [input_velocity_limit_reverse<-900 || ...
          | input_velocity_limit_reverse>0]
      (junction 266) -> (junction 265) [order 2]
      (junction 269) -> (junction 268)
      (junction 265) -> (junction 270) [order 1] : [input_torque_request>350 || ...
          | input_torque_request<-350]
      (junction 265) -> (junction 179) [order 2]
      (junction 270) -> (junction 267)
      (junction 179) -> (junction 180) [order 1] : [1==input_flag_F && 1==input_flag_R]
      (junction 179) -> (junction 181) [order 2]
      (junction 180) -> (junction 185)
      (junction 181) -> (junction 182) [order 1] : [input_accelerator_value < 1.4 || ...
          | input_accelerator_value > 4.5 ]
      (junction 181) -> (junction 183) [order 2]
      (junction 182) -> (junction 184)
      (junction 184) -> (junction 183) : {send(inputs_outside_range, Drive_Mode)}
      (junction 185) -> (junction 184)
      (junction 267) -> (junction 185)
      (junction 268) -> (junction 267)
      (junction 281) -> (junction 268)
      (junction 183) -> (junction 352)
    Input_check_if_statement -> Input_check
  state Fault_check [parallel]
    settings: executionOrder=2
    state Fault_check_if_statement
      (default) -> (junction 255)
      (junction 255) -> (junction 253) [order 1] : [bitand(input_UQM_status(7),uint8(hex2dec('21')))~=0]
      (junction 255) -> (junction 254) [order 2]
      (junction 253) -> (junction 251)
      (junction 254) -> (junction 252) [order 1] : [bitand(input_UQM_status(8),uint8(hex2dec('7E')))~=0]
      (junction 254) -> (junction 239) [order 2]
      (junction 252) -> (junction 250)
      (junction 239) -> (junction 240) [order 1] : [input_UQM_status(5)~=1]
      (junction 239) -> (junction 241) [order 2]
      (junction 240) -> (junction 248)
      (junction 241) -> (junction 242) [order 1] : [input_UQM_status(2)~=0]
      (junction 241) -> (junction 243) [order 2]
      (junction 242) -> (junction 247)
      (junction 243) -> (junction 244) [order 1] : [input_UQM_status(1)~=0]
      (junction 243) -> (junction 245) [order 2]
      (junction 244) -> (junction 246)
      (junction 251) -> (junction 250)
      (junction 250) -> (junction 248)
      (junction 246) -> (junction 245) : {send(FAULT_DETECTED, Drive_Mode)}
      (junction 247) -> (junction 246)
      (junction 248) -> (junction 247)
      (junction 245) -> (junction 249)
    Fault_check_if_statement -> Fault_check
  state FNR_Velocity_Match [parallel]
    settings: executionOrder=3
    state FNR_Velocity_Match_if_statement
      (default) -> (junction 319)
      (junction 319) -> (junction 320) [order 1] : [-5>input_speed && 1==input_flag_F]
      (junction 319) -> (junction 321) [order 2]
      (junction 320) -> (junction 325)
      (junction 321) -> (junction 322) [order 1] : [5<input_speed && 1==input_flag_R]
      (junction 321) -> (junction 323) [order 2] : {FNR_velocity_match_flag=1;}
      (junction 322) -> (junction 324)
      (junction 324) -> (junction 323) : {FNR_velocity_match_flag=0;}
      (junction 325) -> (junction 324)
      (junction 323) -> (junction 326)
    FNR_Velocity_Match_if_statement -> FNR_Velocity_Match
  data: real_val function_input; lower_lim function_input; upper_lim function_input; gain_val function_input; offset_val function_input; output_bytes function_output; input_brake_switch input; input_comms_good_other input boolean; input_steering_mode input; input_speed input; output_chart_state output; input_accelerator_value input; output_fault_lamp output double; input_flag_F input; input_flag_R input; input_UQM_status input uint8 size=8; input_UQM_timeStamp input; input_torque_request input; input_velocity_limit_forward input; input_velocity_limit_reverse input; output_universal_cmd output uint8 size=8; lastUQMWatchDogTime local; universal_cmd_cnt local; FNR_velocity_match_flag local; output_comms_good_self output
  events: FAULT_DETECTED local FUNCTION_CALL_EVENT; inputs_outside_range local FUNCTION_CALL_EVENT; CAN_WD_Timeout local FUNCTION_CALL_EVENT
  function output_bytes = convert_val_to_UQM_CAN_bytes(real_val,lower_lim,upper_lim,gain_val,offset_val):
    | function output_bytes = convert_val_to_UQM_CAN_bytes(real_val,lower_lim,upper_lim,gain_val,offset_val)
    | % saturate the real value between the upper and lower limits
    | real_val = max(real_val,lower_lim);
    | real_val = min(real_val,upper_lim);
    | % convert real value to UQM representation value
    | CAN_val = (round(10*(real_val+offset_val))/10)/gain_val;
    | % cast to uint16 data type
    | CAN_val_int = cast(CAN_val,'uint16');
    | CAN_bytes = typecast(CAN_val_int,'uint8');
    | output_bytes = CAN_bytes(1:2);
    | end
